simulink model "sim_flexible_unsteady_piloted"  (R2018b)
settings: Solver=ode4  StartTime=0.0  StopTime=1000  FixedStep=1/600  RelTol=1e-2  AbsTol=1e-2
model workspace (MAT data in the model file):
  Var = 0
undefined symbols (not defined in the file): aircraft, jystck
libraries: InputBlocks_library x2, se2a_environment_lib x1, flight_dynamics_models x1, aeroelasticity_lib x1, se2a_command_lib x1, joystick_lib x1, dspnetwork x1, flexiFlightVis_lib x1, flightgear_visualization_lib x1, aerolibfltsims x1
settings Model: EnablePacing=on  ParamWorkspaceSource=ReferencedWorkspace  TunableVars=test_val  TunableVarsStorageClass=ExportedGlobal  Creator=Yannic  LastModifiedBy=yannic
settings DataIOCC: ExternalInput=[0,trimPoint.Input']  InitialState=trimPoint.State  LoadExternalInput=on  LoadInitialState=on

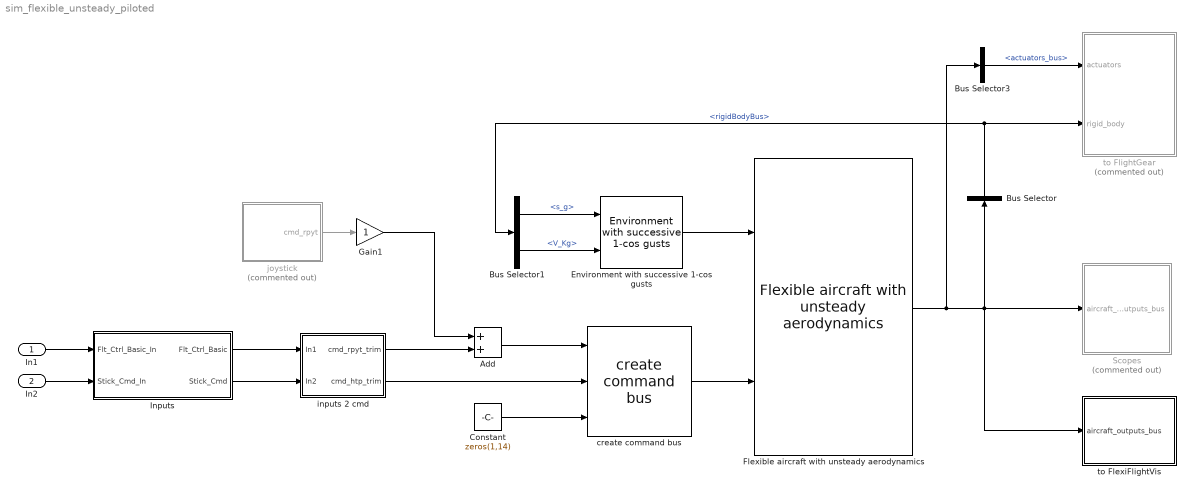
== system sim_flexible_unsteady_piloted ==
  In1 : Inport
  In2 : Inport  Port=2
  Add : Sum
  Bus Selector : BusSelector  OutputSignals=flexible_body_bus.rigidBodyBus
  Bus Selector1 : BusSelector  OutputSignals=s_g,V_Kg
  Bus Selector3 : BusSelector  OutputSignals=actuators_bus
  Constant : Constant  Value=zeros(1,14)
  Environment with successive 1-cos gusts : se2a_environment_lib/Environment with successive 1-cos gusts  envir=envir  pos_ref=pos_ref  wind_input=2  F_g=1  gustGradDist=100  Delta_gustGradDist=10  Delta_time=3  time_0=1
      settings: SourceProductName=SE2A library
  Flexible aircraft with unsteady aerodynamics : flight_dynamics_models/Flexible aircraft with unsteady aerodynamics  aircraft=aircraft  ic=ic
      settings: SourceProductName=SE2A library
  Gain1 : Gain
  Inputs : Subsystem
  Scopes : Subsystem  Commented=on
  create command bus : se2a_command_lib/create command bus  num_ailerons=aircraft.wing_main.params.num_flaps/2
      settings: SourceProductName=SE2A library
  inputs 2 cmd : Subsystem
  joystick : Subsystem  Commented=on
  to FlexiFlightVis : Subsystem
  to FlightGear : Subsystem  Commented=on
  wires:
  Environment with successive 1-cos gusts/1 -> Flexible aircraft with unsteady aerodynamics/1
  create command bus/1 -> Flexible aircraft with unsteady aerodynamics/2
  Bus Selector1/1 -> Environment with successive 1-cos gusts/1  "<s_g>"
  Bus Selector/1 -> to FlightGear/2(rigid_body), Bus Selector1/1  "<rigidBodyBus>"
  Bus Selector1/2 -> Environment with successive 1-cos gusts/2  "<V_Kg>"
  joystick/1(cmd_rpyt) -> Gain1/1
  Flexible aircraft with unsteady aerodynamics/1 -> Bus Selector3/1, to FlexiFlightVis/1(aircraft_outputs_bus), Scopes/1(aircraft_outputs_bus), Bus Selector/1
  Bus Selector3/1 -> to FlightGear/1(actuators)  "<actuators_bus>"
  inputs 2 cmd/2(cmd_htp_trim) -> create command bus/2
  Add/1 -> create command bus/1
  Gain1/1 -> Add/1
  inputs 2 cmd/1(cmd_rpyt_trim) -> Add/2
  Inputs/1(Flt_Ctrl_Basic) -> inputs 2 cmd/1(In1)
  In2/1 -> Inputs/2(Stick_Cmd_In)
  In1/1 -> Inputs/1(Flt_Ctrl_Basic_In)
  Inputs/2(Stick_Cmd) -> inputs 2 cmd/2(In2)
  Constant/1 -> create command bus/3

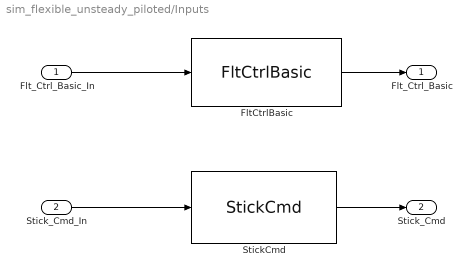
== system sim_flexible_unsteady_piloted/Inputs ==
  Flt_Ctrl_Basic_In : Inport
  Stick_Cmd_In : Inport  Port=2
  FltCtrlBasic : InputBlocks_library/FltCtrlBasic  SystemSampleTime=-1
  StickCmd : InputBlocks_library/StickCmd  SystemSampleTime=-1
  Flt_Ctrl_Basic : Outport
  Stick_Cmd : Outport  Port=2
  wires:
  StickCmd/1 -> Stick_Cmd/1
  FltCtrlBasic/1 -> Flt_Ctrl_Basic/1
  Flt_Ctrl_Basic_In/1 -> FltCtrlBasic/1
  Stick_Cmd_In/1 -> StickCmd/1

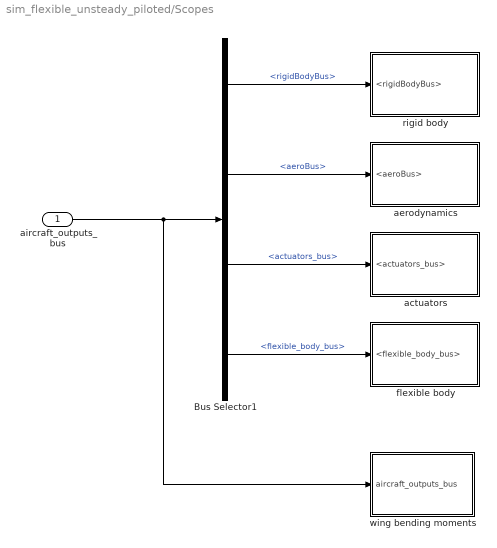
== system sim_flexible_unsteady_piloted/Scopes ==
  aircraft_outputs_bus : Inport
  Bus Selector1 : BusSelector  OutputSignals=flexible_body_bus.rigidBodyBus,aeroBus,actuators_bus,flexible_body_bus
  actuators : Subsystem
  aerodynamics : Subsystem
  flexible body : Subsystem
  rigid body : Subsystem
  wing bending moments : Subsystem
  wires:
  aircraft_outputs_bus/1 -> wing bending moments/1(aircraft_outputs_bus), Bus Selector1/1
  Bus Selector1/1 -> rigid body/1(<rigidBodyBus>)  "<rigidBodyBus>"
  Bus Selector1/2 -> aerodynamics/1(<aeroBus>)  "<aeroBus>"
  Bus Selector1/3 -> actuators/1(<actuators_bus>)  "<actuators_bus>"
  Bus Selector1/4 -> flexible body/1(<flexible_body_bus>)  "<flexible_body_bus>"

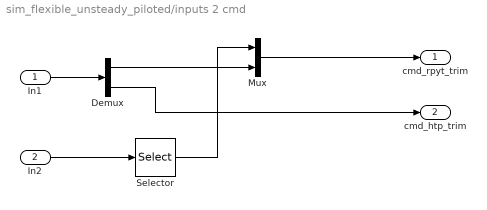
== system sim_flexible_unsteady_piloted/inputs 2 cmd ==
  In1 : Inport
  In2 : Inport  Port=2
  Demux : Demux  Outputs=2
  Mux : Mux  Inputs=2
  Selector : Selector  InputPortWidth=4  IndexOptions=Index vector (dialog)  Indices=1:3  OutputSizes=1
  cmd_rpyt_trim : Outport
  cmd_htp_trim : Outport  Port=2
  wires:
  Demux/1 -> Mux/2
  Selector/1 -> Mux/1
  Mux/1 -> cmd_rpyt_trim/1
  In1/1 -> Demux/1
  Demux/2 -> cmd_htp_trim/1
  In2/1 -> Selector/1

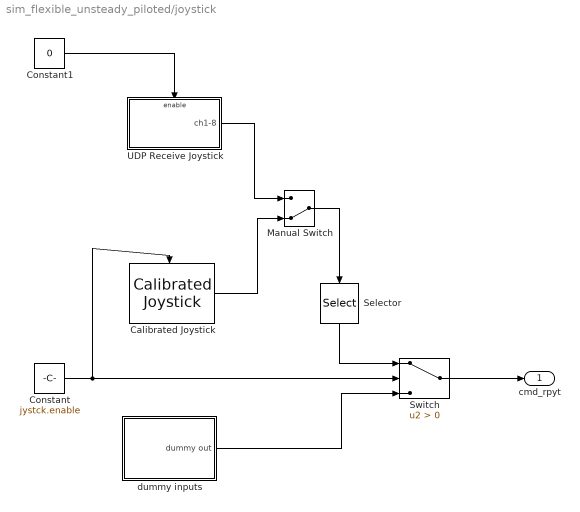
== system sim_flexible_unsteady_piloted/joystick ==
  Calibrated Joystick : joystick_lib/Calibrated Joystick  jystck=joystick  joyid=1
      settings: SourceProductName=LADAC
  Constant : Constant  Value=jystck.enable
  Constant1 : Constant  Value=0
  Manual Switch : ManualSwitch  CurrentSetting=0
  Selector : Selector  InputPortWidth=8  IndexOptions=Index vector (dialog)  Indices=[1,2,3,4]  OutputSizes=1
  Switch : Switch  Criteria=u2 > Threshold
  UDP Receive Joystick : Subsystem
  dummy inputs : Subsystem
  cmd_rpyt : Outport
  wires:
  Switch/1 -> cmd_rpyt/1
  Constant/1 -> Calibrated Joystick/Enable, Switch/2
  dummy inputs/1(dummy out) -> Switch/3
  Selector/1 -> Switch/1
  UDP Receive Joystick/1(ch1-8) -> Manual Switch/1
  Manual Switch/1 -> Selector/1
  Calibrated Joystick/1 -> Manual Switch/2
  Constant1/1 -> UDP Receive Joystick/Enable

== system sim_flexible_unsteady_piloted/to FlexiFlightVis ==
  aircraft_outputs_bus : Inport
  Bus Creator : BusCreator  Inputs=1
  Bus Selector : BusSelector  OutputSignals=flexible_body_bus.rigidBodyBus,aeroBus.main,aeroBus.htp,aeroBus.vtp,aeroBus.fuselage
  Constant1 : Constant  Value=aircraft.config.xyz_ref_c  VectorParams1D=off
  Send to FlexiFlightVis : flexiFlightVis_lib/Send to FlexiFlightVis  sample_time=1/60  ip_address='localhost'  ip_port=4321  wing_cell={aircraft.wing_main.state,aircraft.wing_htp.state,aircraft.wing_vtp.state}  fuse_cell={aircraft.fuselage.state}
      settings: SourceProductName=LADAC
  wires:
  aircraft_outputs_bus/1 -> Bus Selector/1
  Bus Selector/1 -> Send to FlexiFlightVis/1  "<rigidBodyBus>"
  Bus Selector/2 -> Send to FlexiFlightVis/3  "<main>"
  Bus Selector/3 -> Send to FlexiFlightVis/4  "<htp>"
  Bus Selector/4 -> Send to FlexiFlightVis/5  "<vtp>"
  Constant1/1 -> Bus Creator/1  "xyz_ref_c"
  Bus Creator/1 -> Send to FlexiFlightVis/2  "config"
  Bus Selector/5 -> Send to FlexiFlightVis/6  "<fuselage>"

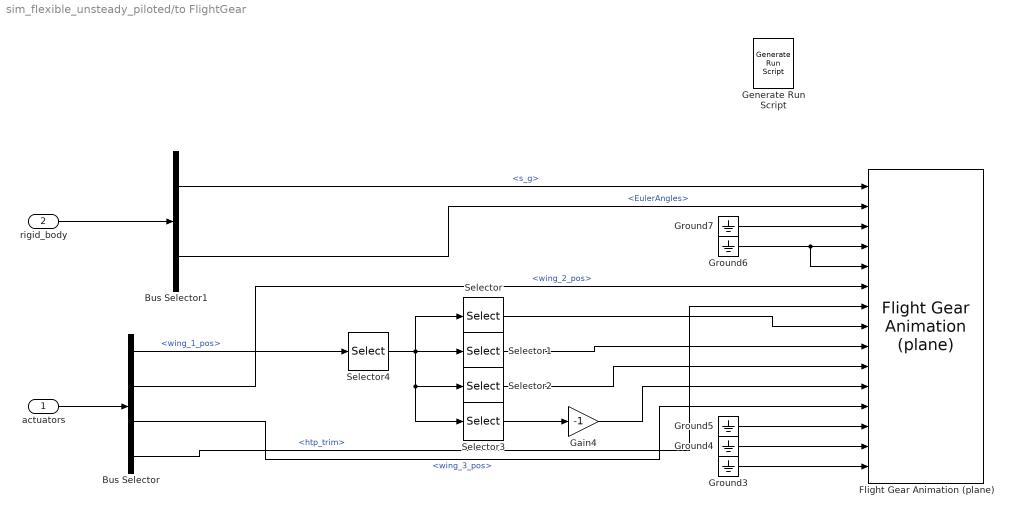
== system sim_flexible_unsteady_piloted/to FlightGear ==
  actuators : Inport
  rigid_body : Inport  Port=2
  Bus Selector : BusSelector  OutputSignals=wing_1_pos,wing_2_pos,wing_3_pos,htp_trim
  Bus Selector1 : BusSelector  OutputSignals=s_g,EulerAngles
  Flight Gear Animation (plane) : flightgear_visualization_lib/Flight Gear Animation (plane)  inital_lat=pos_ref.lat  inital_long=pos_ref.lon  inital_height=pos_ref.alt  remoteURL='127.0.0.1'  remotePort=5502
      settings: SourceProductName=LADAC
  Gain4 : Gain  Gain=-1
  Generate Run Script : aerolibfltsims/Generate Run Script  Architecture=Win64  dataFlow=Send  GeometryModelName=777  AirportId=KSFO  RunwayId=10L  InitialAltitude=7224  InitialHeading=113  OffsetDistance=4.72  OffsetAzimuth=0  InstallScenery=off  DisableShaders=off  OriginAddress=127.0.0.1  DestinationPort=5502  OriginPort=5505  LocalAddress=127.0.0.1  OutputFileName=runfg.bat  FlightGearBaseDirectory=C:\Program Files\FlightGear 3.4.0
  Ground{3..7} (5 alike) : Ground
  Selector : Selector  InputPortWidth=6  IndexOptions=Index vector (dialog)  Indices=3  OutputSizes=1
  Selector1 : Selector  InputPortWidth=6  IndexOptions=Index vector (dialog)  Indices=4  OutputSizes=1
  Selector2 : Selector  InputPortWidth=6  IndexOptions=Index vector (dialog)  Indices=1  OutputSizes=1
  Selector3 : Selector  InputPortWidth=6  IndexOptions=Index vector (dialog)  Indices=6  OutputSizes=1
  Selector4 : Selector  InputPortWidth=20  IndexOptions=Index vector (dialog)  Indices=[1:6]  OutputSizes=1
  wires:
  Bus Selector1/2 -> Flight Gear Animation (plane)/2  "<EulerAngles>"
  Bus Selector1/1 -> Flight Gear Animation (plane)/1  "<s_g>"
  Bus Selector/3 -> Flight Gear Animation (plane)/12  "<wing_3_pos>"
  Selector4/1 -> Selector2/1, Selector3/1, Selector/1, Selector1/1
  Selector/1 -> Flight Gear Animation (plane)/8
  Selector1/1 -> Flight Gear Animation (plane)/9
  Selector2/1 -> Flight Gear Animation (plane)/10
  Selector3/1 -> Gain4/1
  Gain4/1 -> Flight Gear Animation (plane)/11
  actuators/1 -> Bus Selector/1
  Bus Selector/1 -> Selector4/1  "<wing_1_pos>"
  Bus Selector/2 -> Flight Gear Animation (plane)/6  "<wing_2_pos>"
  Bus Selector/4 -> Flight Gear Animation (plane)/7  "<htp_trim>"
  rigid_body/1 -> Bus Selector1/1
  Ground5/1 -> Flight Gear Animation (plane)/13
  Ground4/1 -> Flight Gear Animation (plane)/14
  Ground3/1 -> Flight Gear Animation (plane)/15
  Ground6/1 -> Flight Gear Animation (plane)/5, Flight Gear Animation (plane)/4
  Ground7/1 -> Flight Gear Animation (plane)/3

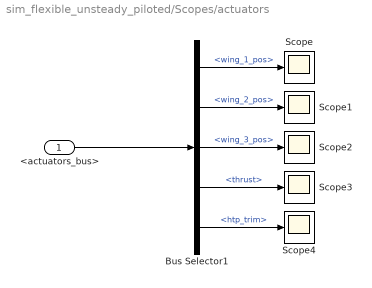
== system sim_flexible_unsteady_piloted/Scopes/actuators ==
  <actuators_bus> : Inport
  Bus Selector1 : BusSelector  OutputSignals=wing_1_pos,wing_2_pos,wing_3_pos,thrust,htp_trim
  Scope{,1..4} (5 alike) : Scope
  wires:
  <actuators_bus>/1 -> Bus Selector1/1
  Bus Selector1/1 -> Scope/1  "<wing_1_pos>"
  Bus Selector1/2 -> Scope1/1  "<wing_2_pos>"
  Bus Selector1/3 -> Scope2/1  "<wing_3_pos>"
  Bus Selector1/4 -> Scope3/1  "<thrust>"
  Bus Selector1/5 -> Scope4/1  "<htp_trim>"

== system sim_flexible_unsteady_piloted/Scopes/aerodynamics ==
  <aeroBus> : Inport
  Bus Selector1 : BusSelector  OutputSignals=main,htp,vtp
  htp : Subsystem
  vtp : Subsystem
  wing : Subsystem
  wires:
  <aeroBus>/1 -> Bus Selector1/1
  Bus Selector1/2 -> htp/1(htp)  "<htp>"
  Bus Selector1/1 -> wing/1(main)  "<main>"
  Bus Selector1/3 -> vtp/1(vtp)  "<vtp>"

== system sim_flexible_unsteady_piloted/Scopes/flexible body ==
  <flexible_body_bus> : Inport
  Bus Selector1 : BusSelector  OutputSignals=eta,eta_dt,eta_dt2,generalized_load_vector
  Scope{,1..3} (4 alike) : Scope
  wires:
  Bus Selector1/4 -> Scope3/1  "<generalized_load_vector>"
  Bus Selector1/3 -> Scope2/1  "<eta_dt2>"
  Bus Selector1/2 -> Scope1/1  "<eta_dt>"
  Bus Selector1/1 -> Scope/1  "<eta>"
  <flexible_body_bus>/1 -> Bus Selector1/1

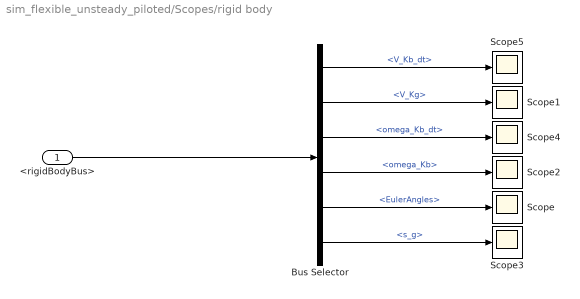
== system sim_flexible_unsteady_piloted/Scopes/rigid body ==
  <rigidBodyBus> : Inport
  Bus Selector : BusSelector  OutputSignals=V_Kb_dt,V_Kg,omega_Kb_dt,omega_Kb,EulerAngles,s_g
  Scope{,1..5} (6 alike) : Scope
  wires:
  Bus Selector/5 -> Scope/1  "<EulerAngles>"
  Bus Selector/2 -> Scope1/1  "<V_Kg>"
  Bus Selector/6 -> Scope3/1  "<s_g>"
  Bus Selector/4 -> Scope2/1  "<omega_Kb>"
  <rigidBodyBus>/1 -> Bus Selector/1
  Bus Selector/3 -> Scope4/1  "<omega_Kb_dt>"
  Bus Selector/1 -> Scope5/1  "<V_Kb_dt>"

== system sim_flexible_unsteady_piloted/Scopes/wing bending moments ==
  aircraft_outputs_bus : Inport
  Bus Selector4 : BusSelector  OutputSignals=flexible_body_bus.eta
  Scope : Scope
  wing dynamic bending moment1 : aeroelasticity_lib/wing dynamic bending moment  structure=structure  structure_red=aircraft.eom_flexible.structure_red  eta=[-0.9:0.2:0.9]
      settings: SourceProductName=LADAC
  wires:
  Bus Selector4/1 -> wing dynamic bending moment1/1  "<eta>"
  aircraft_outputs_bus/1 -> Bus Selector4/1
  wing dynamic bending moment1/1 -> Scope/1

== system sim_flexible_unsteady_piloted/joystick/UDP Receive Joystick ==
  Enable : EnablePort
  Terminator : Terminator
  UDP Receive1 : dspnetwork/UDP Receive  localURL='0.0.0.0'  localPort=25000  remoteURL='192.168.178.2'  remotePort=-1  recvBufferSize=8*8  dims=8  signalDatatype=double  isVarSize=off  showBlockingTime=on  blockingTime=1  sampletime=1/30  blockPlatform=HOST
      settings: SourceProductName=DSP System Toolbox  SourceProductBaseCode=DS
  ch1-8 : Outport
  wires:
  UDP Receive1/1 -> ch1-8/1
  UDP Receive1/2 -> Terminator/1

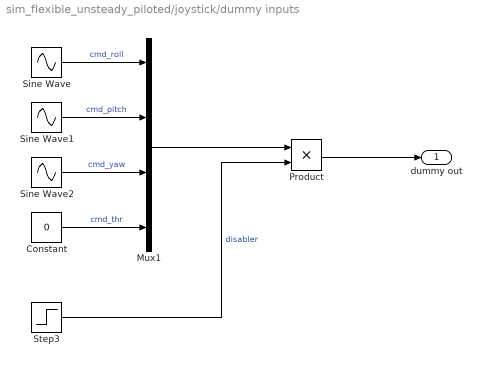
== system sim_flexible_unsteady_piloted/joystick/dummy inputs ==
  Constant : Constant  Value=0
  Mux1 : Mux
  Product : Product
  Sine Wave : Sin  Amplitude=0.1  Frequency=3  SampleTime=0
  Sine Wave1 : Sin  Amplitude=0.1  Frequency=4  SampleTime=0
  Sine Wave2 : Sin  Amplitude=0.1  Frequency=5  SampleTime=0
  Step3 : Step  Time=10  Before=1  After=0  SampleTime=0
  dummy out : Outport
  wires:
  Constant/1 -> Mux1/4  "cmd_thr"
  Sine Wave2/1 -> Mux1/3  "cmd_yaw"
  Sine Wave1/1 -> Mux1/2  "cmd_pitch"
  Sine Wave/1 -> Mux1/1  "cmd_roll"
  Mux1/1 -> Product/1
  Product/1 -> dummy out/1
  Step3/1 -> Product/2  "disabler"

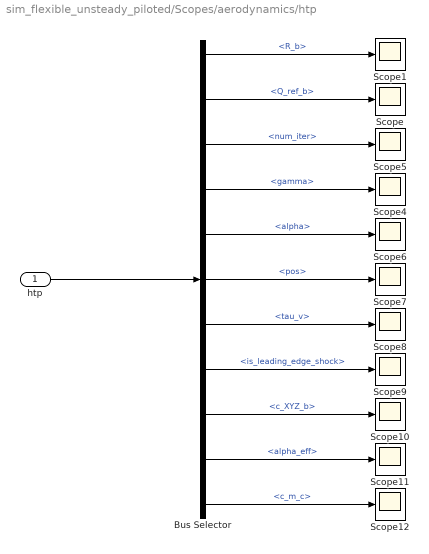
== system sim_flexible_unsteady_piloted/Scopes/aerodynamics/htp ==
  htp : Inport
  Bus Selector : BusSelector  OutputSignals=aero.force_glob.R_b,aero.force_glob.Q_ref_b,aero.circulation.num_iter,aero.circulation.gamma,body.alpha,actuators.pos,aero.unsteady.tau_v,aero.unsteady.is_leading_edge_shock,aero.coeff_loc.c_XYZ_b,aero.circulation.alpha_eff,aero.unsteady.c_m_c
  Scope{,1,4..12} (11 alike) : Scope
  wires:
  Bus Selector/11 -> Scope12/1  "<c_m_c>"
  Bus Selector/10 -> Scope11/1  "<alpha_eff>"
  Bus Selector/9 -> Scope10/1  "<c_XYZ_b>"
  Bus Selector/8 -> Scope9/1  "<is_leading_edge_shock>"
  Bus Selector/7 -> Scope8/1  "<tau_v>"
  Bus Selector/6 -> Scope7/1  "<pos>"
  Bus Selector/5 -> Scope6/1  "<alpha>"
  htp/1 -> Bus Selector/1
  Bus Selector/1 -> Scope1/1  "<R_b>"
  Bus Selector/2 -> Scope/1  "<Q_ref_b>"
  Bus Selector/4 -> Scope4/1  "<gamma>"
  Bus Selector/3 -> Scope5/1  "<num_iter>"

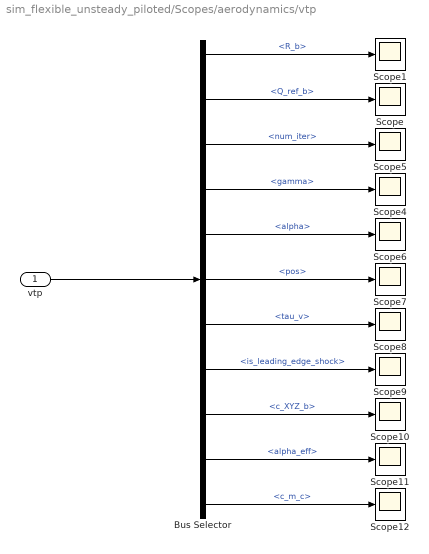
== system sim_flexible_unsteady_piloted/Scopes/aerodynamics/vtp ==
  vtp : Inport
  Bus Selector : BusSelector  OutputSignals=aero.force_glob.R_b,aero.force_glob.Q_ref_b,aero.circulation.num_iter,aero.circulation.gamma,body.alpha,actuators.pos,aero.unsteady.tau_v,aero.unsteady.is_leading_edge_shock,aero.coeff_loc.c_XYZ_b,aero.circulation.alpha_eff,aero.unsteady.c_m_c
  Scope{,1,4..12} (11 alike) : Scope
  wires:
  Bus Selector/3 -> Scope5/1  "<num_iter>"
  Bus Selector/4 -> Scope4/1  "<gamma>"
  Bus Selector/2 -> Scope/1  "<Q_ref_b>"
  Bus Selector/1 -> Scope1/1  "<R_b>"
  vtp/1 -> Bus Selector/1
  Bus Selector/5 -> Scope6/1  "<alpha>"
  Bus Selector/6 -> Scope7/1  "<pos>"
  Bus Selector/7 -> Scope8/1  "<tau_v>"
  Bus Selector/8 -> Scope9/1  "<is_leading_edge_shock>"
  Bus Selector/9 -> Scope10/1  "<c_XYZ_b>"
  Bus Selector/10 -> Scope11/1  "<alpha_eff>"
  Bus Selector/11 -> Scope12/1  "<c_m_c>"

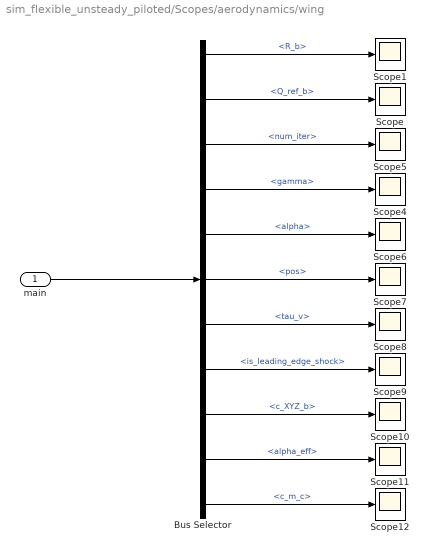
== system sim_flexible_unsteady_piloted/Scopes/aerodynamics/wing ==
  main : Inport
  Bus Selector : BusSelector  OutputSignals=aero.force_glob.R_b,aero.force_glob.Q_ref_b,aero.circulation.num_iter,aero.circulation.gamma,body.alpha,actuators.pos,aero.unsteady.tau_v,aero.unsteady.is_leading_edge_shock,aero.coeff_loc.c_XYZ_b,aero.circulation.alpha_eff,aero.unsteady.c_m_c
  Scope{,1,4..12} (11 alike) : Scope
  wires:
  Bus Selector/3 -> Scope5/1  "<num_iter>"
  Bus Selector/4 -> Scope4/1  "<gamma>"
  Bus Selector/2 -> Scope/1  "<Q_ref_b>"
  Bus Selector/1 -> Scope1/1  "<R_b>"
  main/1 -> Bus Selector/1
  Bus Selector/5 -> Scope6/1  "<alpha>"
  Bus Selector/6 -> Scope7/1  "<pos>"
  Bus Selector/7 -> Scope8/1  "<tau_v>"
  Bus Selector/8 -> Scope9/1  "<is_leading_edge_shock>"
  Bus Selector/9 -> Scope10/1  "<c_XYZ_b>"
  Bus Selector/10 -> Scope11/1  "<alpha_eff>"
  Bus Selector/11 -> Scope12/1  "<c_m_c>"
